simulink model "EjemploPioneer2"  (Simulink 7.6)
settings: Solver=FixedStepDiscrete  StartTime=0.0  StopTime=inf  FixedStep=0.01  RelTol=1e-3
libraries: simulink x2, aerolibanimutils x1
settings Model: Creator=Usuario  LastModifiedBy=Usuario

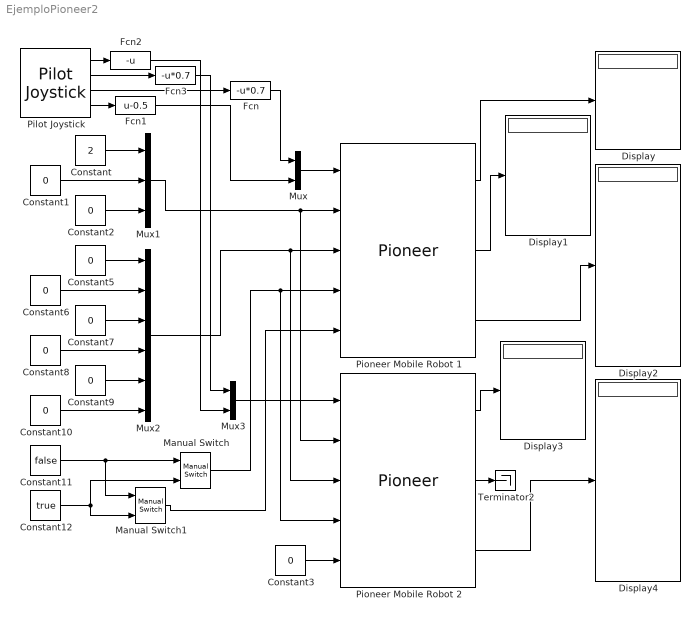
== system EjemploPioneer2 ==
  Constant : Constant  Value=2
  Constant1 : Constant  Value=0
  Constant{5..10} (6 alike) : Constant  Value=0  OutDataTypeStr=int32
  Constant11 : Constant  Value=false
  Constant12 : Constant  Value=true
  Constant2 : Constant  Value=0
  Constant3 : Constant  Value=0  OutDataTypeStr=boolean
  Display{,1..4} (5 alike) : Display
  Fcn : Fcn  Expr=-u*0.7
  Fcn1 : Fcn  Expr=u-0.5
  Fcn2 : Fcn  Expr=-u
  Fcn3 : Fcn  Expr=-u*0.7
  Manual Switch : simulink/Signal Routing/Manual Switch  SystemSampleTime=-1  sw=1  action=0  varsize=off
  Manual Switch1 : simulink/Signal Routing/Manual Switch  SystemSampleTime=-1  sw=1  action=0  varsize=off
  Mux : Mux  Inputs=2
  Mux1 : Mux  Inputs=3
  Mux2 : Mux  Inputs=6
  Mux3 : Mux  Inputs=2
  Pilot Joystick : aerolibanimutils/Pilot Joystick  JoystickID=Joystick1  OutputConfiguration=FourAxis  SampleTime=0.01
  Pioneer Mobile Robot 1 : S-Function  FunctionName=Pioneer  Parameters=1  EnableBusSupport=off
      mask Display:
      | color('red')
      | port_label('input',1,'acciones')
      | port_label('input',2,'postura')
      | port_label('input',3,'parametros')
      | port_label('input',4,'parametrosSend')
      | port_label('input',5,'posturaSend')
      | color('blue')
      | port_label('output',1,'estado')
      | port_label('output',2,'parametros')
      | port_label('output',3,'laser')
  Pioneer Mobile Robot 2 : S-Function  FunctionName=Pioneer  Parameters=2  EnableBusSupport=off
      mask Display:
      | color('red')
      | port_label('input',1,'acciones')
      | port_label('input',2,'postura')
      | port_label('input',3,'parametros')
      | port_label('input',4,'parametrosSend')
      | port_label('input',5,'posturaSend')
      | color('blue')
      | port_label('output',1,'estado')
      | port_label('output',2,'parametros')
      | port_label('output',3,'laser')
  Terminator2 : Terminator
  wires:
  Pilot Joystick/3 -> Fcn/1
  Pilot Joystick/4 -> Fcn1/1
  Mux/1 -> Pioneer Mobile Robot 1/1
  Fcn/1 -> Mux/1
  Fcn1/1 -> Mux/2
  Constant/1 -> Mux1/1
  Constant1/1 -> Mux1/2
  Constant2/1 -> Mux1/3
  Constant5/1 -> Mux2/1
  Constant6/1 -> Mux2/2
  Constant7/1 -> Mux2/3
  Constant8/1 -> Mux2/4
  Constant9/1 -> Mux2/5
  Constant10/1 -> Mux2/6
  Constant11/1 -> Manual Switch/1, Manual Switch1/1
  Constant12/1 -> Manual Switch/2, Manual Switch1/2
  Manual Switch1/1 -> Pioneer Mobile Robot 1/5
  Mux1/1 -> Pioneer Mobile Robot 1/2, Pioneer Mobile Robot 2/2
  Mux2/1 -> Pioneer Mobile Robot 1/3, Pioneer Mobile Robot 2/3
  Pioneer Mobile Robot 1/2 -> Display1/1
  Pioneer Mobile Robot 1/1 -> Display/1
  Pioneer Mobile Robot 1/3 -> Display2/1
  Pioneer Mobile Robot 2/1 -> Display3/1
  Pioneer Mobile Robot 2/2 -> Terminator2/1
  Pioneer Mobile Robot 2/3 -> Display4/1
  Manual Switch/1 -> Pioneer Mobile Robot 1/4, Pioneer Mobile Robot 2/4
  Mux3/1 -> Pioneer Mobile Robot 2/1
  Pilot Joystick/2 -> Fcn3/1
  Pilot Joystick/1 -> Fcn2/1
  Fcn2/1 -> Mux3/2
  Fcn3/1 -> Mux3/1
  Constant3/1 -> Pioneer Mobile Robot 2/5
